simulink model "Check_TF"  (R2014b)
settings: Solver=ode45  StartTime=0.0  StopTime=20  RelTol=1e-3
libraries: simulink x1
settings Model: Creator=Asus  LastModifiedBy=Asus

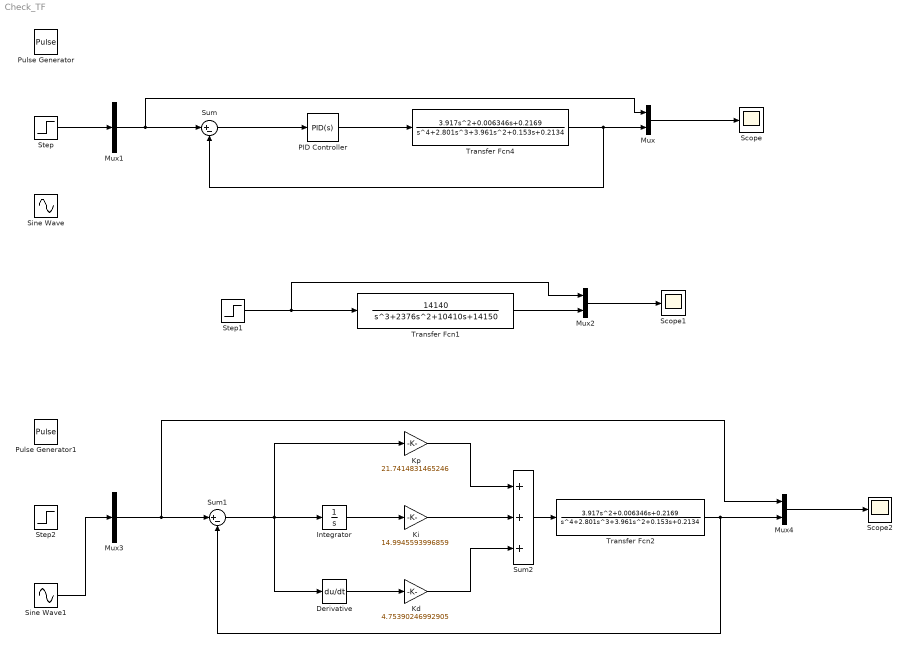
== system Check_TF ==
  Derivative : Derivative
  Integrator : Integrator
  Kd : Gain  Gain=4.75390246992905
  Ki : Gain  Gain=14.9945593996859
  Kp : Gain  Gain=21.7414831465246
  Mux : Mux  Inputs=2
  Mux1 : Mux  Inputs=1
  Mux2 : Mux  Inputs=2
  Mux3 : Mux  Inputs=1
  Mux4 : Mux  Inputs=2
  PID Controller : simulink/Continuous/PID Controller  Controller=PID  TimeDomain=Continuous-time  SampleTime=-1  IntegratorMethod=Forward Euler  FilterMethod=Forward Euler  Form=Parallel  P=21.7414831465246  I=14.9945593996859  D=4.75390246992905  N=106.029452778944  InitialConditionSource=internal  InitialConditionForIntegrator=0  InitialConditionForFilter=0  ExternalReset=none  LimitOutput=off  UpperSaturationLimit=inf  LowerSaturationLimit=-inf  LinearizeAsGain=on  AntiWindupMode=none  Kb=1  TrackingMode=off  Kt=1  PParamMin=[]  PParamMax=[]  IParamMin=[]  IParamMax=[]  DParamMin=[]  DParamMax=[]  NParamMin=[]  NParamMax=[]  KbParamMin=[]  KbParamMax=[]  KtParamMin=[]  KtParamMax=[]  POutMin=[]  POutMax=[]  IOutMin=[]  IOutMax=[]  DOutMin=[]  DOutMax=[]  NOutMin=[]  NOutMax=[]  KbOutMin=[]  KbOutMax=[]  KtOutMin=[]  KtOutMax=[]  IntegratorOutMin=[]  IntegratorOutMax=[]  FilterOutMin=[]  FilterOutMax=[]  SumOutMin=[]  SumOutMax=[]  SumI1OutMin=[]  SumI1OutMax=[]  SumI2OutMin=[]  SumI2OutMax=[]  SumI3OutMin=[]  SumI3OutMax=[]  SumDOutMin=[]  SumDOutMax=[]  SaturationOutMin=[]  SaturationOutMax=[]  IntegratorContinuousStateAttributes=''  IntegratorStateMustResolveToSignalObject=off  IntegratorRTWStateStorageClass=Auto  FilterContinuousStateAttributes=''  FilterStateMustResolveToSignalObject=off  FilterRTWStateStorageClass=Auto  DifferentiatorICPrevScaledInput=0  DifferentiatorOutMin=[]  DifferentiatorOutMax=[]  UseFilter=on
  Pulse Generator : DiscretePulseGenerator  PulseType=Time based  Period=4  PulseWidth=50
  Pulse Generator1 : DiscretePulseGenerator  PulseType=Time based  Period=4  PulseWidth=50
  Scope : Scope
      settings: ShowLegends=on
  Scope1 : Scope
      settings: ShowLegends=on
  Scope2 : Scope
      settings: ShowLegends=on  SaveName=ScopeData2
  Sine Wave : Sin  SampleTime=0
  Sine Wave1 : Sin  SampleTime=0
  Step : Step  SampleTime=0
  Step1 : Step  SampleTime=0
  Step2 : Step  SampleTime=0
  Sum : Sum  Inputs=|+-
  Sum1 : Sum  Inputs=|+-
  Sum2 : Sum  Inputs=+++
  Transfer Fcn1 : TransferFcn  Numerator=[14140]  Denominator=[1 2376 10410 14150]
  Transfer Fcn2 : TransferFcn  Numerator=[3.917 0.006346 0.2169]  Denominator=[1 2.801 3.961 0.153 0.2134]
  Transfer Fcn4 : TransferFcn  Numerator=[3.917 0.006346 0.2169]  Denominator=[1 2.801 3.961 0.153 0.2134]
  wires:
  Sum/1 -> PID Controller/1
  PID Controller/1 -> Transfer Fcn4/1
  Transfer Fcn4/1 -> Sum/2, Mux/2
  Mux/1 -> Scope/1
  Mux1/1 -> Mux/1, Sum/1
  Step1/1 -> Mux2/1, Transfer Fcn1/1
  Transfer Fcn1/1 -> Mux2/2
  Mux2/1 -> Scope1/1
  Mux3/1 -> Mux4/1, Sum1/1
  Sum1/1 -> Derivative/1, Integrator/1, Kp/1
  Integrator/1 -> Ki/1
  Derivative/1 -> Kd/1
  Kp/1 -> Sum2/1
  Ki/1 -> Sum2/2
  Kd/1 -> Sum2/3
  Sum2/1 -> Transfer Fcn2/1
  Mux4/1 -> Scope2/1
  Transfer Fcn2/1 -> Mux4/2, Sum1/2
  Sine Wave1/1 -> Mux3/1
  Step/1 -> Mux1/1
